simulink model "pos_8mot"  (R2021a)
settings: Solver=FixedStepDiscrete  StartTime=0.0  StopTime=inf  FixedStep=0.001  RelTol=1e-3  EnableMultiTasking=on
InitFcn:
  | load("rho_CommandCalib.mat");
  | run("importCmd.m")
model workspace (MAT data in the model file):
  positionCmd = [145.742 145.741 145.741 145.74 145.74 145.739 145.738 145.738 145.737 145.737 145.736 145.735 ... (560000 elements, 70000x8)]
  tempsTraj = [25 25 20]
values from neighbouring files (symbols this model uses):
  rho_CommandCalib = [325.033 325.033 325.033 325.033 325.033 325.033 325.033 325.033 325.033 325.033 325.033 325.033 ... (80000 elements, 10000x8)]    [rho_CommandCalib.mat]
undefined symbols (not defined in the file or in its folder): rho_CommandCircXY, rho_CommandCroixTilt, rho_CommandCroixXY, rho_CommandInclinaison, rho_CommandInclinaisonInterieure, rho_CommandPickAndPlace, rho_CommandPickAndPlaceTilt, rho_CommandPickAndPlaceVertical, rho_CommandPickAndPlaceX, rho_CommandSinusZ, rho_CommandSinusZ_decentree, rho_CommandTwist
libraries: xpcethercatlib x64, slrealtimeethercatlib x36, commutil2 x19, slrealtimeobsoletelib x7
(part 2 of 3)

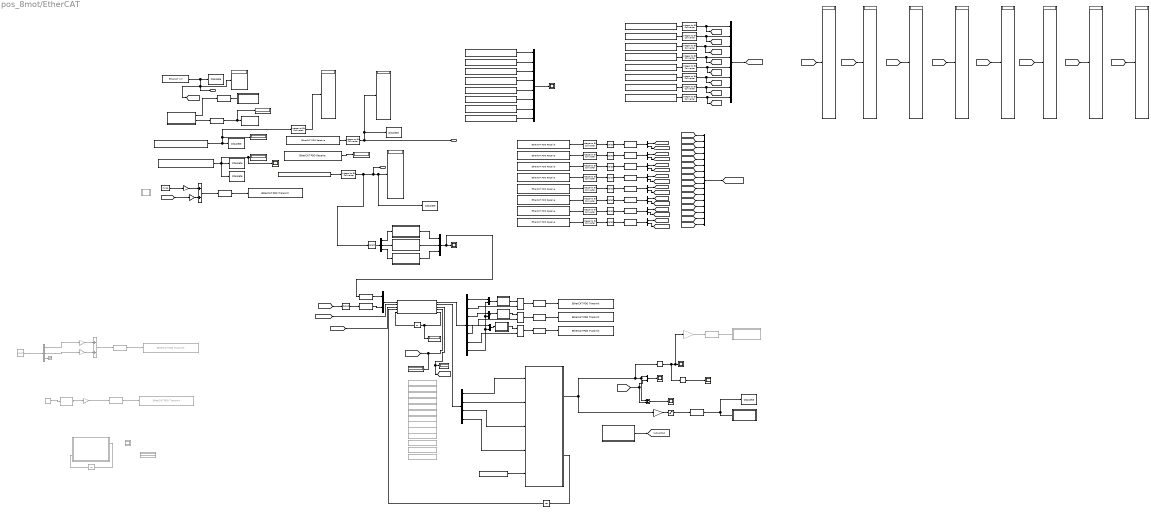
== system pos_8mot/EtherCAT ==
  note: Stand alone : PCI Bus 0 Slot 25, Otherwise : PCI Bus 3 Slot 0
  note: LinMot Warning Word
  note: Status Word from LinMot Drive
  note: Machine d'état
  note: Gestion des lumières
  note: Gestion des boutons
  note: Test 1 lumière clignotante
  note: Test 2 boutons 1 lumière
  note: Operation Enabled
      | Switch on Active
      | Operation Enabled
      | Fault
      | Voltage Enabled
      | Quick Stop
      | Switch on disabled
      | Warning
      | event Handler Active
      | Special Motion Active
      | Target Reached
      | Homed
      | Fatal Error
      | Motion Active
      | Range Indicator 1
      | Range Indicator 2
  note: 4688 = Standby
      | 4663 = Ready to go!!!
      | 536 = Fault
      | 4657 = Fault reset
  note: Set control word
  note: Operation Enabled
      | Switch on Active
      | Enable Operation
      | Fault
      | Voltage Enabled
      | Quick Stop
      | Switch on disabled
      | Warning
      | event Handler Active
      | Special Motion Active
      | Target Reached
      | Homed
      | Fatal Error
      | Motion Active
      | Range Indicator 1
      | Range Indicator 2
  note: Digital In X4.5
      | Digital In X4.6
      | Digital In X4.7
      | Digital In X4.8
      | Forced Bit Mask
      | Forced Bit Mask
      | empty
      | empty
      | empty
      | empty
      | empty
      | empty
      | empty
      | empty
      | empty
      | empty
  Activation1 : Subsystem
  Actual Motor Position : Subsystem
  Add : Sum
  Add1 : Sum  Commented=on
  Alimentation : Subsystem  Commented=on
      settings: OpenFcn=|
      | if strcmp(get_param([gcb '/Manual Switch'], 'sw'), '1')
      |   set_param([gcb '/Manual Switch'], 'sw', '0');
      |   set_param(gcb, 'MaskDisplay', 'fprintf(''ON'')','BackgroundColor','green');
      | else
      |   set_param([gcb '/Manual Switch'], 'sw', '1');
      |   set_param(gcb, 'MaskDisplay', 'fprintf(''OFF'')','BackgroundColor','red');
      | end
      mask Display: fprintf('OFF')
  Cast To Double{2..9} (8 alike) : DataTypeConversion  OutDataTypeStr=double
  Commande et réelle : Scope
  Constant : Constant  Commented=on  Value=[0.5 0]
  Constant1 : Constant  Commented=on  Value=rho_CommandPickAndPlace
  Constant10 : Constant  Commented=on  Value=rho_CommandInclinaisonInterieure
  Constant11 : Constant  Commented=on  Value=rho_CommandTwist
  Constant18 : Constant  Commented=on  Value=rho_CommandCalib
  Constant19 : Constant  Value=rho_CommandCalib
  Constant2 : Constant  Commented=on  Value=rho_CommandCroixTilt
  Constant21 : Constant  Commented=on  Value=rho_CommandSinusZ_decentree
  Constant22 : Constant  Commented=on  Value=rho_CommandPickAndPlaceVertical
  Constant3 : Constant  Commented=on  Value=rho_CommandPickAndPlaceX
  Constant4 : Constant  Commented=on  Value=rho_CommandSinusZ
  Constant5 : Constant  Commented=on  Value=rho_CommandCircXY
  Constant6 : Constant  Commented=on  Value=rho_CommandCroixXY
  Constant7 : Constant  Commented=on  Value=rho_CommandInclinaison
  Constant8 : Constant  Commented=on  Value=rho_CommandPickAndPlaceTilt
  Current Drive 1 : slrealtimeethercatlib/EtherCAT PDO Receive  Priority=2  sig_name=Drive 1 (C1150-DS-XC-0S).Cylic Mode Inputs.DemandCurrent  sig_offset=776  sig_type=int32  type_size=32  sig_dim=1  device_id=0  sample_time=0.001000
      settings: SourceProductBaseCode=XP
  Current Drive 10 : slrealtimeethercatlib/EtherCAT PDO Receive  Priority=2  sig_name=Drive 2 (C1150-DS-XC-0S).User Defined Inputs.Warn Word LinMot  sig_offset=1016  sig_type=uint16  type_size=16  sig_dim=1  device_id=0  sample_time=0.001000
      settings: SourceProductBaseCode=XP
  Current Drive 11 : slrealtimeethercatlib/EtherCAT PDO Receive  Priority=2  sig_name=Drive 3 (C1150-DS-XC-0S).User Defined Inputs.Warn Word LinMot  sig_offset=1176  sig_type=uint16  type_size=16  sig_dim=1  device_id=0  sample_time=0.001000
      settings: SourceProductBaseCode=XP
  Current Drive 12 : slrealtimeethercatlib/EtherCAT PDO Receive  Priority=2  sig_name=Drive 4 (C1150-DS-XC-0S).User Defined Inputs.Warn Word LinMot  sig_offset=1336  sig_type=uint16  type_size=16  sig_dim=1  device_id=0  sample_time=0.001000
      settings: SourceProductBaseCode=XP
  Current Drive 13 : slrealtimeethercatlib/EtherCAT PDO Receive  Priority=2  sig_name=Drive 5 (C1150-DS-XC-0S).User Defined Inputs.Warn Word LinMot  sig_offset=1496  sig_type=uint16  type_size=16  sig_dim=1  device_id=0  sample_time=0.001000
      settings: SourceProductBaseCode=XP
  Current Drive 14 : slrealtimeethercatlib/EtherCAT PDO Receive  Priority=2  sig_name=Drive 6 (C1150-DS-XC-0S).User Defined Inputs.Warn Word LinMot  sig_offset=1656  sig_type=uint16  type_size=16  sig_dim=1  device_id=0  sample_time=0.001000
      settings: SourceProductBaseCode=XP
  Current Drive 15 : slrealtimeethercatlib/EtherCAT PDO Receive  Priority=2  sig_name=Drive 7 (C1150-DS-XC-0S).User Defined Inputs.Warn Word LinMot  sig_offset=1816  sig_type=uint16  type_size=16  sig_dim=1  device_id=0  sample_time=0.001000
      settings: SourceProductBaseCode=XP
  Current Drive 16 : slrealtimeethercatlib/EtherCAT PDO Receive  Priority=2  sig_name=Drive 8 (C1150-DS-XC-0S).User Defined Inputs.Warn Word LinMot  sig_offset=1976  sig_type=uint16  type_size=16  sig_dim=1  device_id=0  sample_time=0.001000
      settings: SourceProductBaseCode=XP
  Current Drive 2 : slrealtimeethercatlib/EtherCAT PDO Receive  Priority=2  sig_name=Drive 2 (C1150-DS-XC-0S).Cylic Mode Inputs.DemandCurrent  sig_offset=952  sig_type=int32  type_size=32  sig_dim=1  device_id=0  sample_time=0.001000
      settings: SourceProductBaseCode=XP
  Current Drive 3 : slrealtimeethercatlib/EtherCAT PDO Receive  Priority=2  sig_name=Drive 3 (C1150-DS-XC-0S).Cylic Mode Inputs.DemandCurrent  sig_offset=1112  sig_type=int32  type_size=32  sig_dim=1  device_id=0  sample_time=0.001000
      settings: SourceProductBaseCode=XP
  Current Drive 4 : slrealtimeethercatlib/EtherCAT PDO Receive  Priority=2  sig_name=Drive 4 (C1150-DS-XC-0S).Cylic Mode Inputs.DemandCurrent  sig_offset=1272  sig_type=int32  type_size=32  sig_dim=1  device_id=0  sample_time=0.001000
      settings: SourceProductBaseCode=XP
  Current Drive 5 : slrealtimeethercatlib/EtherCAT PDO Receive  Priority=2  sig_name=Drive 5 (C1150-DS-XC-0S).Cylic Mode Inputs.DemandCurrent  sig_offset=1432  sig_type=int32  type_size=32  sig_dim=1  device_id=0  sample_time=0.001000
      settings: SourceProductBaseCode=XP
  Current Drive 6 : slrealtimeethercatlib/EtherCAT PDO Receive  Priority=2  sig_name=Drive 6 (C1150-DS-XC-0S).Cylic Mode Inputs.DemandCurrent  sig_offset=1592  sig_type=int32  type_size=32  sig_dim=1  device_id=0  sample_time=0.001000
      settings: SourceProductBaseCode=XP
  Current Drive 7 : slrealtimeethercatlib/EtherCAT PDO Receive  Priority=2  sig_name=Drive 7 (C1150-DS-XC-0S).Cylic Mode Inputs.DemandCurrent  sig_offset=1752  sig_type=int32  type_size=32  sig_dim=1  device_id=0  sample_time=0.001000
      settings: SourceProductBaseCode=XP
  Current Drive 8 : slrealtimeethercatlib/EtherCAT PDO Receive  Priority=2  sig_name=Drive 8 (C1150-DS-XC-0S).Cylic Mode Inputs.DemandCurrent  sig_offset=1912  sig_type=int32  type_size=32  sig_dim=1  device_id=0  sample_time=0.001000
      settings: SourceProductBaseCode=XP
  Current Drive 9 : slrealtimeethercatlib/EtherCAT PDO Receive  Priority=2  sig_name=Drive 1 (C1150-DS-XC-0S).User Defined Inputs.Warn Word LinMot  sig_offset=856  sig_type=uint16  type_size=16  sig_dim=1  device_id=0  sample_time=0.001000
      settings: SourceProductBaseCode=XP
  Data Type Conversion : DataTypeConversion  OutDataTypeStr=int32
  Data Type Conversion{1,3,8..10} (5 alike) : DataTypeConversion  OutDataTypeStr=uint16
  Data Type Conversion11 : DataTypeConversion  Commented=on  OutDataTypeStr=int32
  Data Type Conversion2 : DataTypeConversion  OutDataTypeStr=int8
  Data Type Conversion4 : DataTypeConversion  Commented=on  OutDataTypeStr=uint16
  Data Type Conversion5 : DataTypeConversion  Commented=on  OutDataTypeStr=uint16
  Data Type Conversion6 : DataTypeConversion  OutDataTypeStr=double
  Data Type Conversion7 : DataTypeConversion  OutDataTypeStr=double
  Demux : Demux  Commented=on  Outputs=3
  Demux1 : Demux  Outputs=3
  Demux{4..11} (8 alike) : Demux  Outputs=2
  Demux2 : Demux  Outputs=7
  Demux3 : Demux
  Digital In Word form Linmot UPID : slrealtimeethercatlib/EtherCAT PDO Receive  Priority=2  sig_name=Drive 1 (C1150-DS-XC-0S).User Defined Inputs.Digital Input Word  sig_offset=824  sig_type=uint16  type_size=16  sig_dim=1  device_id=0  sample_time=0.001000
      settings: SourceProductBaseCode=XP
  Digital Output Word : slrealtimeethercatlib/EtherCAT PDO Transmit  Priority=3  sig_name=Drive 1 (C1150-DS-XC-0S).User Defined Outputs.Digital Output Word  sig_offset=760  sig_type=uint16  type_size=16  sig_dim=1  device_id=0  sample_time=0.001000
      settings: SourceProductBaseCode=XP
  Digital Output Word1 : slrealtimeethercatlib/EtherCAT PDO Transmit  Priority=3  Commented=on  sig_name=Drive 2 (C1150-DS-XC-0S).User Defined Outputs.Digital Output Word  sig_offset=920  sig_type=uint16  type_size=16  sig_dim=1  device_id=0  sample_time=0.001000
      settings: SourceProductBaseCode=XP
  Digital Output Word2 : slrealtimeethercatlib/EtherCAT PDO Transmit  Priority=3  Commented=on  sig_name=Drive 2 (C1150-DS-XC-0S).User Defined Outputs.Digital Output Word  sig_offset=920  sig_type=uint16  type_size=16  sig_dim=1  device_id=0  sample_time=0.001000
      settings: SourceProductBaseCode=XP
  Digital Output Word3 : slrealtimeethercatlib/EtherCAT PDO Transmit  Priority=3  sig_name=Drive 2 (C1150-DS-XC-0S).User Defined Outputs.Digital Output Word  sig_offset=936  sig_type=uint16  type_size=16  sig_dim=1  device_id=0  sample_time=0.001000
      settings: SourceProductBaseCode=XP
  Digital Output Word4 : slrealtimeethercatlib/EtherCAT PDO Transmit  Priority=3  sig_name=Drive 3 (C1150-DS-XC-0S).User Defined Outputs.Digital Output Word  sig_offset=1096  sig_type=uint16  type_size=16  sig_dim=1  device_id=0  sample_time=0.001000
      settings: SourceProductBaseCode=XP
  Digital Output Word5 : slrealtimeethercatlib/EtherCAT PDO Transmit  Priority=3  sig_name=Drive 4 (C1150-DS-XC-0S).User Defined Outputs.Digital Output Word  sig_offset=1256  sig_type=uint16  type_size=16  sig_dim=1  device_id=0  sample_time=0.001000
      settings: SourceProductBaseCode=XP
  Display{,1..4,6..14} (14 alike) : Display
  Display5 : Display  Commented=on
  Erreur : Scope
  "EtherCAT Init " : slrealtimeethercatlib/EtherCAT Init  Priority=0  config_file=U:\Maitrise\Planification de trajectoire\TwinCAT\8motor_pos_control_IO\8mot_poscont_IO_ENI_V2.xml  device_id=0  pci_bus=0  pci_slot=0  pci_function=0  portnum=1  initstate=2  dctuning=0  enaDebug=0  enaDC=on  errLink=off  masterDbg=off  stateChgDbg=off  baseClock=off  masterCfg=off  logFile='c:\dbglog.txt'  sample_time=0.001000  DCMode=2
      settings: SourceProductBaseCode=XP
  Gain : Gain  Gain=2^0
  Gain1 : Gain  Gain=2^1
  Gain2 : Gain  Commented=on  Gain=2^0
  Gain3 : Gain  Commented=on  Gain=2^1
  Gain4 : Gain  Commented=on  Gain=2^0
  Integer to Bit Converter{,1..18} (19 alike) : commutil2/Integer to Bit Converter  nbits=16  signedInputValues=Unsigned  bitOrder=LSB first  outDtype=Inherit via internal rule
  LOG_Acceleration : Derivative
  LOG_Current : Mux  Inputs=8
  LOG_Erreur : Sum  Inputs=+-
  LOG_Vitesse : Derivative
  MATLAB Function : MATLAB Function  Commented=on  TreatAsAtomicUnit=on
  MATLAB Function1 : MATLAB Function  TreatAsAtomicUnit=on
  MATLAB Function2 : MATLAB Function  Commented=on  TreatAsAtomicUnit=on
  MATLAB Function3 : MATLAB Function  TreatAsAtomicUnit=on
  MATLAB Function4 : MATLAB Function  TreatAsAtomicUnit=on
  MATLAB Function5 : MATLAB Function  TreatAsAtomicUnit=on
  MATLAB Function6 : MATLAB Function  TreatAsAtomicUnit=on
  MATLAB Function7 : MATLAB Function  TreatAsAtomicUnit=on
  MATLAB Function8 : MATLAB Function  TreatAsAtomicUnit=on
  MATLAB Function9 : MATLAB Function  TreatAsAtomicUnit=on
  Matrix Multiply : Product  Multiplication=Matrix(*)
  Matrix Multiply1 : Product  Multiplication=Matrix(*)
  Matrix Multiply2 : Product  Multiplication=Matrix(*)
  Mode : Display
  Mode Selection : Display
  Mode of Operation Display : slrealtimeethercatlib/EtherCAT PDO Receive  Priority=2  sig_name=Drive 7 (C1150-DS-XC-0S).Cylic Mode Inputs.Mode of Operation display  sig_offset=1784  sig_type=int8  type_size=8  sig_dim=1  device_id=0  sample_time=0.001000
      settings: SourceProductBaseCode=XP
  Mux : Mux  Inputs=3
  Mux{1..5} (5 alike) : Mux  Inputs=2
  Mux8 : Mux  Inputs=16
  Position : Display
  Position Actual Value : slrealtimeethercatlib/EtherCAT PDO Receive  Priority=2  sig_name=Drive 7 (C1150-DS-XC-0S).Cylic Mode Inputs.Position actual value (units)  sig_offset=1688  sig_type=int32  type_size=32  sig_dim=1  device_id=0  sample_time=0.001000
      settings: SourceProductBaseCode=XP
  Pulse WatchDog : DiscretePulseGenerator  PulseType=Time based  Period=0.1  PulseWidth=50
  Saturation1 : Saturate  UpperLimit=3250000  LowerLimit=10000
  Scope : Scope  Commented=on
  Scope Position : Scope
  "Scope " : slrealtimeobsoletelib/Obsolete  ObsoleteBlock=slrtlib/Displays and Logging/Scope  ObsoleteParameters=|  NumInports=1  NumOutports=0
      | ContentPreviewEnabled:  off
      | scopeno:  1
      | scopetype:  Target
      | autostart:  on
      | viewmode:  Numerical
      | formatstr:  '%6.0f,%6.0f,%6.0f,%6.0f,%6.0f,%6.0f'
      | grid:  on
      | ylimits:  [0,0]
      | nosamples:  3
      | noprepostsamples:  0
      | interleave:  1
      | triggermode:  FreeRun
      | triggersignal:  1
      | trigsignalfromport:  off
      | triggerlevel:  0.0
      | triggerslope:  Either
      | triggerscope:  1
      | triggersample:  0
      | filename:  data.dat
      | mode:  Lazy
      | writesize:  512
      | autorestart:  off
      | dynamicfilemode:  off
      | maxwritefilesize:  512*1024^2
      settings: SourceProductBaseCode=XP
  Scope 1 : slrealtimeobsoletelib/Obsolete  ObsoleteBlock=slrtlib/Displays and Logging/Scope  ObsoleteParameters=|  NumInports=1  NumOutports=0
      | ContentPreviewEnabled:  off
      | scopeno:  3
      | scopetype:  Target
      | autostart:  on
      | viewmode:  Numerical
      | formatstr:  '%15.6f'
      | grid:  on
      | ylimits:  [0,0]
      | nosamples:  3
      | noprepostsamples:  0
      | interleave:  1
      | triggermode:  FreeRun
      | triggersignal:  1
      | trigsignalfromport:  off
      | triggerlevel:  0.0
      | triggerslope:  Either
      | triggerscope:  1
      | triggersample:  0
      | filename:  data.dat
      | mode:  Lazy
      | writesize:  512
      | autorestart:  off
      | dynamicfilemode:  off
      | maxwritefilesize:  512*1024^2
      settings: SourceProductBaseCode=XP
  Scope 2 : slrealtimeobsoletelib/Obsolete  ObsoleteBlock=slrtlib/Displays and Logging/Scope  ObsoleteParameters=|  NumInports=1  NumOutports=0
      | ContentPreviewEnabled:  off
      | scopeno:  4
      | scopetype:  Target
      | autostart:  on
      | viewmode:  Graphical sliding
      | formatstr:  '%15.6f'
      | grid:  on
      | ylimits:  [-1000000,1000000]
      | nosamples:  2000
      | noprepostsamples:  0
      | interleave:  1
      | triggermode:  FreeRun
      | triggersignal:  1
      | trigsignalfromport:  off
      | triggerlevel:  0.0
      | triggerslope:  Either
      | triggerscope:  1
      | triggersample:  0
      | filename:  data.dat
      | mode:  Lazy
      | writesize:  512
      | autorestart:  off
      | dynamicfilemode:  off
      | maxwritefilesize:  512*1024^2
      settings: SourceProductBaseCode=XP
  Scope 3 : slrealtimeobsoletelib/Obsolete  ObsoleteBlock=slrtlib/Displays and Logging/Scope  ObsoleteParameters=|  NumInports=1  NumOutports=0
      | ContentPreviewEnabled:  off
      | scopeno:  2
      | scopetype:  Target
      | autostart:  on
      | viewmode:  Graphical sliding
      | formatstr:  '%15.6f'
      | grid:  on
      | ylimits:  [0,0]
      | nosamples:  1000
      | noprepostsamples:  0
      | interleave:  1
      | triggermode:  FreeRun
      | triggersignal:  1
      | trigsignalfromport:  off
      | triggerlevel:  0.0
      | triggerslope:  Either
      | triggerscope:  1
      | triggersample:  0
      | filename:  data.dat
      | mode:  Lazy
      | writesize:  512
      | autorestart:  off
      | dynamicfilemode:  off
      | maxwritefilesize:  512*1024^2
      settings: SourceProductBaseCode=XP
  Scope 4 : slrealtimeobsoletelib/Obsolete  ObsoleteBlock=slrtlib/Displays and Logging/Scope  ObsoleteParameters=|  NumInports=1  NumOutports=0
      | ContentPreviewEnabled:  off
      | scopeno:  5
      | scopetype:  Target
      | autostart:  on
      | viewmode:  Numerical
      | formatstr:  '%15.6f'
      | grid:  on
      | ylimits:  [0,0]
      | nosamples:  3
      | noprepostsamples:  0
      | interleave:  1
      | triggermode:  FreeRun
      | triggersignal:  1
      | trigsignalfromport:  off
      | triggerlevel:  0.0
      | triggerslope:  Either
      | triggerscope:  1
      | triggersample:  0
      | filename:  data.dat
      | mode:  Lazy
      | writesize:  512
      | autorestart:  off
      | dynamicfilemode:  off
      | maxwritefilesize:  512*1024^2
      settings: SourceProductBaseCode=XP
  Scope 5 : slrealtimeobsoletelib/Obsolete  ObsoleteBlock=slrtlib/Displays and Logging/Scope  ObsoleteParameters=|  NumInports=1  NumOutports=0
      | ContentPreviewEnabled:  off
      | scopeno:  6
      | scopetype:  Target
      | autostart:  on
      | viewmode:  Numerical
      | formatstr:  'Digital In X4.5 %1.0f, Digital In X4.6 %1.0f, Digital In X4.7 %1.0f, Digital In X4.8 %1.0f, Forced Bit Mask %1.0f, Forced Bit Mask %1.0f'
      | grid:  on
      | ylimits:  [0,0]
      | nosamples:  3
      | noprepostsamples:  0
      | interleave:  1
      | triggermode:  FreeRun
      | triggersignal:  1
      | trigsignalfromport:  off
      | triggerlevel:  0.0
      | triggerslope:  Either
      | triggerscope:  1
      | triggersample:  0
      | filename:  data.dat
      | mode:  Lazy
      | writesize:  512
      | autorestart:  off
      | dynamicfilemode:  off
      | maxwritefilesize:  512*1024^2
      settings: SourceProductBaseCode=XP
  Scope 6 : slrealtimeobsoletelib/Obsolete  ObsoleteBlock=slrtlib/Displays and Logging/Scope  ObsoleteParameters=|  NumInports=1  NumOutports=0
      | ContentPreviewEnabled:  off
      | scopeno:  7
      | scopetype:  Target
      | autostart:  on
      | viewmode:  Numerical
      | formatstr:  'Operation Enabled %1.0f, Switch on Active %1.0f, Enable Operation %1.0f, Fault %1.0f, Voltage Enabled %1.0f, Quick Stop %1.0f, Switch on disabled %1.0f, Warning %1.0f, event Handler Active %1.0f, Special Motion Active %1.0f, target Reached %1.0f, Homed %1.0f, Fatal Error %1.0f, Motion Active %1.0f, Range Indicator 1 %1.0f, Range Indicator 2 %1.0f'
      | grid:  on
      | ylimits:  [0,0]
      | nosamples:  3
      | noprepostsamples:  0
      | interleave:  1
      | triggermode:  FreeRun
      | triggersignal:  1
      | trigsignalfromport:  off
      | triggerlevel:  0.0
      | triggerslope:  Either
      | triggerscope:  1
      | triggersample:  0
      | filename:  data.dat
      | mode:  Lazy
      | writesize:  512
      | autorestart:  off
      | dynamicfilemode:  off
      | maxwritefilesize:  512*1024^2
      settings: SourceProductBaseCode=XP
  Scope{1..2,4..5} (4 alike) : Scope
  Selector : Selector  Commented=on  InputPortWidth=16  IndexOptions=Index vector (dialog)  Indices=[1 2 3]  OutputSizes=1
  Selector1 : Selector  InputPortWidth=16  IndexOptions=Index vector (dialog)  Indices=[1 2 3]  OutputSizes=1
  Selector{4..11} (8 alike) : Selector  InputPortWidth=16  IndexOptions=Index vector (dialog)  Indices=[4 12]  OutputSizes=1
  Selector2 : Selector  InputPortWidth=6  IndexOptions=Index vector (dialog)  Indices=[2]  OutputSizes=1
  Send Control Word : Subsystem
  Send Position : Subsystem
  Send mode of opreation : Subsystem
  Send velocity : Subsystem  Commented=on
  State : Display
  StatuWord from Linmot UPID : slrealtimeethercatlib/EtherCAT PDO Receive  Priority=2  sig_name=Drive 7 (C1150-DS-XC-0S).User Defined Inputs.StatusWord Linmot  sig_offset=1800  sig_type=uint16  type_size=16  sig_dim=1  device_id=0  sample_time=0.001000
      settings: SourceProductBaseCode=XP
  StatuWord from Linmot UPID1 : slrealtimeethercatlib/EtherCAT PDO Receive  Priority=2  sig_name=Drive 1 (C1150-DS-XC-0S).User Defined Inputs.StatusWord Linmot  sig_offset=840  sig_type=uint16  type_size=16  sig_dim=1  device_id=0  sample_time=0.001000
      settings: SourceProductBaseCode=XP
  StatuWord from Linmot UPID2 : slrealtimeethercatlib/EtherCAT PDO Receive  Priority=2  sig_name=Drive 2 (C1150-DS-XC-0S).User Defined Inputs.StatusWord Linmot  sig_offset=1000  sig_type=uint16  type_size=16  sig_dim=1  device_id=0  sample_time=0.001000
      settings: SourceProductBaseCode=XP
  StatuWord from Linmot UPID3 : slrealtimeethercatlib/EtherCAT PDO Receive  Priority=2  sig_name=Drive 3 (C1150-DS-XC-0S).User Defined Inputs.StatusWord Linmot  sig_offset=1160  sig_type=uint16  type_size=16  sig_dim=1  device_id=0  sample_time=0.001000
      settings: SourceProductBaseCode=XP
  StatuWord from Linmot UPID4 : slrealtimeethercatlib/EtherCAT PDO Receive  Priority=2  sig_name=Drive 4 (C1150-DS-XC-0S).User Defined Inputs.StatusWord Linmot  sig_offset=1320  sig_type=uint16  type_size=16  sig_dim=1  device_id=0  sample_time=0.001000
      settings: SourceProductBaseCode=XP
  StatuWord from Linmot UPID5 : slrealtimeethercatlib/EtherCAT PDO Receive  Priority=2  sig_name=Drive 5 (C1150-DS-XC-0S).User Defined Inputs.StatusWord Linmot  sig_offset=1480  sig_type=uint16  type_size=16  sig_dim=1  device_id=0  sample_time=0.001000
      settings: SourceProductBaseCode=XP
  StatuWord from Linmot UPID6 : slrealtimeethercatlib/EtherCAT PDO Receive  Priority=2  sig_name=Drive 6 (C1150-DS-XC-0S).User Defined Inputs.StatusWord Linmot  sig_offset=1640  sig_type=uint16  type_size=16  sig_dim=1  device_id=0  sample_time=0.001000
      settings: SourceProductBaseCode=XP
  StatuWord from Linmot UPID7 : slrealtimeethercatlib/EtherCAT PDO Receive  Priority=2  sig_name=Drive 7 (C1150-DS-XC-0S).User Defined Inputs.StatusWord Linmot  sig_offset=1800  sig_type=uint16  type_size=16  sig_dim=1  device_id=0  sample_time=0.001000
      settings: SourceProductBaseCode=XP
  StatuWord from Linmot UPID8 : slrealtimeethercatlib/EtherCAT PDO Receive  Priority=2  sig_name=Drive 8 (C1150-DS-XC-0S).User Defined Inputs.StatusWord Linmot  sig_offset=1960  sig_type=uint16  type_size=16  sig_dim=1  device_id=0  sample_time=0.001000
      settings: SourceProductBaseCode=XP
  StatusWord : slrealtimeethercatlib/EtherCAT PDO Receive  Priority=2  sig_name=Drive 7 (C1150-DS-XC-0S).Cylic Mode Inputs.Statusword  sig_offset=1672  sig_type=uint16  type_size=16  sig_dim=1  device_id=0  sample_time=0.001000
      settings: SourceProductBaseCode=XP
  Terminator : Terminator  Commented=on
  Unit Delay : UnitDelay  Commented=on  SampleTime=-1  HasFrameUpgradeWarning=on
  Unit Delay1 : UnitDelay  SampleTime=-1  HasFrameUpgradeWarning=on
  Unit Delay2 : UnitDelay  SampleTime=-1  HasFrameUpgradeWarning=on
  Vector Concatenate : Concatenate  NumInputs=8  Mode=Multidimensional array  ConcatenateDimension=2
  mm to um : Gain  Commented=on  Gain=10000
  signaux : Display
  to linmot unit : Gain  Gain=10000
  ECAT_status : Outport
  SW_linmot : Outport  Port=2
  Digital_IN : Outport  Port=3
  tag scope: modeSelection=global
  wires:
  Activation1/2(ControlWord) -> Data Type Conversion1/1
  Data Type Conversion1/1 -> Send Control Word/1(In1), Display2/1
  Data Type Conversion/1 -> Send Position/1(Commanded Position), Scope 3/1  "Commanded Position"
  StatusWord/1 -> Integer to Bit Converter/1, Display/1, Scope 1/1  "Status word"
  Position Actual Value/1 -> Scope 4/1, Scope Position/1, Position/1, Scope 2/1  "Actual Position"
  Saturation1/1 -> Data Type Conversion/1
  Mode of Operation Display/1 -> Mode/1  "Status word"
  Integer to Bit Converter/1 -> Display3/1
  to linmot unit/1 -> Saturation1/1
  Digital In Word form Linmot UPID/1 -> Integer to Bit Converter1/1  "digital"
  Integer to Bit Converter1/1 -> Selector1/1, Digital_IN/1, Scope 5/1, signaux/1
  StatuWord from Linmot UPID/1 -> Integer to Bit Converter2/1  "bouton"
  Integer to Bit Converter2/1 -> SW_linmot/1, Scope 6/1, Display4/1
  Gain1/1 -> Add/2
  Gain/1 -> Add/1
  Pulse WatchDog/1 -> Gain/1
  Add/1 -> Data Type Conversion3/1
  Data Type Conversion3/1 -> Digital Output Word/1
  Data Type Conversion2/1 -> Send mode of opreation/1(In1)
  Activation1/1(mode of operation) -> Data Type Conversion2/1
  Data Type Conversion4/1 -> Digital Output Word1/1
  Demux/2 -> Gain3/1
  Gain2/1 -> Add1/1
  Gain3/1 -> Add1/2
  Demux/1 -> Gain2/1
  Add1/1 -> Data Type Conversion4/1
  Selector/1 -> Demux/1
  Demux/3 -> Terminator/1
  MATLAB Function/1(y) -> Gain4/1
  Gain4/1 -> Data Type Conversion5/1
  Data Type Conversion5/1 -> Digital Output Word2/1
  MATLAB Function2/1(new_state) -> Unit Delay/1
  Unit Delay/1 -> MATLAB Function2/2(state)
  Mux/1 -> Data Type Conversion7/1, Scope1/1
  MATLAB Function1/1(isPressed) -> Mux/1
  MATLAB Function3/1(isPressed) -> Mux/2
  MATLAB Function4/1(isPressed) -> Mux/3
  Selector1/1 -> Demux1/1
  Demux1/2 -> MATLAB Function3/1(buttonState)
  Demux1/1 -> MATLAB Function1/1(buttonState)
  Demux1/3 -> MATLAB Function4/1(buttonState)
  "EtherCAT Init "/1 -> [ECAT_Status], ECAT_status/1, Display1/1, "Scope "/1
  [ECAT_Status] -> Selector2/1
  Mux1/1 -> MATLAB Function5/1(inputs)
  MATLAB Function5/5(new_state) -> State/1, Unit Delay1/1
  Unit Delay1/1 -> MATLAB Function5/5(state)
  Selector2/1 -> Data Type Conversion6/1
  Data Type Conversion6/1 -> Mux1/2
  Data Type Conversion7/1 -> Mux1/1
  Data Type Conversion10/1 -> Digital Output Word5/1
  Data Type Conversion9/1 -> Digital Output Word4/1
  Data Type Conversion8/1 -> Digital Output Word3/1
  Matrix Multiply2/1 -> Data Type Conversion8/1
  Matrix Multiply1/1 -> Data Type Conversion9/1
  Matrix Multiply/1 -> Data Type Conversion10/1
  MATLAB Function5/1(outputs_LED) -> Demux2/1
  Constant/1 -> MATLAB Function/1(u)
  MATLAB Function8/1(y) -> Matrix Multiply/1
  MATLAB Function7/1(y) -> Matrix Multiply1/1
  MATLAB Function6/1(y) -> Matrix Multiply2/1
  Demux2/2 -> Matrix Multiply2/2
  Demux2/4 -> Matrix Multiply1/2
  Demux2/6 -> Matrix Multiply/2
  Demux2/1 -> Mux2/1
  Demux2/3 -> Mux3/1
  Demux2/5 -> Mux4/1
  Mux2/1 -> MATLAB Function6/1(u)
  Demux2/7 -> Mux4/2, Mux3/2, Mux2/2
  Mux4/1 -> MATLAB Function8/1(u)
  Mux3/1 -> MATLAB Function7/1(u)
  MATLAB Function5/2(outputs_traj) -> Demux3/1
  MATLAB Function5/3(selectionMode) -> [modeSelection], Mode Selection/1
  Demux3/1 -> MATLAB Function9/1(trajectorySelector)
  Demux3/2 -> MATLAB Function9/2(pause)
  Demux3/3 -> MATLAB Function9/3(stopAtEnd)
  Demux3/4 -> MATLAB Function9/4(waitForActivation)
  Constant19/1 -> MATLAB Function9/5(position_from_gabarit_to_standby)
  MATLAB Function9/2(isCompleted) -> Unit Delay2/1
  Unit Delay2/1 -> MATLAB Function5/4(isCompleted)
  Mux5/1 -> Commande et réelle/1
  LOG_Erreur/1 -> Erreur/1
  [ActualPos] -> Mux5/2, LOG_Erreur/2
  MATLAB Function5/4(motorPower) -> Display6/1, [motorPower]
  [StatusWord_LinMot] -> MATLAB Function5/2(statusWordLinMot)
  [motorPower] -> Gain1/1
  MATLAB Function9/1(target) -> LOG_Vitesse/1, Mux5/1, LOG_Erreur/1, to linmot unit/1
  Actual Motor Position/1(Actual Position) -> [ActualPos]
  Current Drive 8/1 -> LOG_Current/8
  Current Drive 6/1 -> LOG_Current/6
  Current Drive 7/1 -> LOG_Current/7
  Current Drive 5/1 -> LOG_Current/5
  Current Drive 4/1 -> LOG_Current/4
  Current Drive 3/1 -> LOG_Current/3
  Current Drive 2/1 -> LOG_Current/2
  Current Drive 1/1 -> LOG_Current/1
  LOG_Current/1 -> Scope4/1
  LOG_Vitesse/1 -> LOG_Acceleration/1, mm to um/1, Scope5/1
  Data Type Conversion11/1 -> Send velocity/1(Command velocity)  "Commanded Velocity"
  mm to um/1 -> Data Type Conversion11/1
  LOG_Acceleration/1 -> Scope2/1
  StatuWord from Linmot UPID1/1 -> Integer to Bit Converter3/1  "bouton"
  StatuWord from Linmot UPID2/1 -> Integer to Bit Converter4/1  "bouton"
  StatuWord from Linmot UPID3/1 -> Integer to Bit Converter5/1  "bouton"
  StatuWord from Linmot UPID4/1 -> Integer to Bit Converter6/1  "bouton"
  StatuWord from Linmot UPID5/1 -> Integer to Bit Converter7/1  "bouton"
  StatuWord from Linmot UPID6/1 -> Integer to Bit Converter8/1  "bouton"
  StatuWord from Linmot UPID7/1 -> Integer to Bit Converter9/1  "bouton"
  StatuWord from Linmot UPID8/1 -> Integer to Bit Converter10/1  "bouton"
  Selector4/1 -> Cast To Double2/1
  Selector5/1 -> Cast To Double3/1
  Selector6/1 -> Cast To Double4/1
  Selector7/1 -> Cast To Double5/1
  Selector8/1 -> Cast To Double6/1
  Selector9/1 -> Cast To Double7/1
  Selector10/1 -> Cast To Double8/1
  Selector11/1 -> Cast To Double9/1
  Integer to Bit Converter3/1 -> Selector4/1
  Integer to Bit Converter4/1 -> Selector5/1
  Integer to Bit Converter5/1 -> Selector6/1
  Integer to Bit Converter6/1 -> Selector7/1
  Integer to Bit Converter7/1 -> Selector8/1
  Integer to Bit Converter8/1 -> Selector9/1
  Integer to Bit Converter9/1 -> Selector10/1
  Integer to Bit Converter10/1 -> Selector11/1
  Cast To Double2/1 -> Demux4/1
  Cast To Double3/1 -> Demux5/1
  Cast To Double4/1 -> Demux6/1
  Cast To Double5/1 -> Demux7/1
  Cast To Double6/1 -> Demux8/1
  Cast To Double7/1 -> Demux9/1
  Cast To Double8/1 -> Demux10/1
  Cast To Double9/1 -> Demux11/1
  Demux4/1 -> [faultDrive1]
  Demux4/2 -> [isHomedDrive1]
  Demux5/1 -> [faultDrive2]
  Demux5/2 -> [isHomedDrive2]
  Demux6/1 -> [faultDrive3]
  Demux6/2 -> [isHomedDrive3]
  Demux7/1 -> [faultDrive4]
  Demux7/2 -> [isHomedDrive4]
  Demux8/1 -> [faultDrive5]
  Demux8/2 -> [isHomedDrive5]
  Demux9/1 -> [faultDrive6]
  Demux9/2 -> [isHomedDrive6]
  Demux10/1 -> [faultDrive7]
  Demux10/2 -> [isHomedDrive7]
  Demux11/1 -> [faultDrive8]
  Demux11/2 -> [isHomedDrive8]
  [faultDrive6] -> Mux8/6
  [faultDrive1] -> Mux8/1
  [faultDrive2] -> Mux8/2
  [faultDrive3] -> Mux8/3
  [faultDrive4] -> Mux8/4
  [faultDrive5] -> Mux8/5
  [faultDrive7] -> Mux8/7
  [faultDrive8] -> Mux8/8
  [isHomedDrive1] -> Mux8/9
  [isHomedDrive2] -> Mux8/10
  [isHomedDrive3] -> Mux8/11
  [isHomedDrive4] -> Mux8/12
  [isHomedDrive5] -> Mux8/13
  [isHomedDrive6] -> Mux8/14
  [isHomedDrive7] -> Mux8/15
  [isHomedDrive8] -> Mux8/16
  Mux8/1 -> [StatusWord_LinMot]
  Current Drive 9/1 -> Integer to Bit Converter11/1
  Current Drive 10/1 -> Integer to Bit Converter12/1
  Current Drive 11/1 -> Integer to Bit Converter13/1
  Current Drive 12/1 -> Integer to Bit Converter14/1
  Current Drive 13/1 -> Integer to Bit Converter15/1
  Current Drive 14/1 -> Integer to Bit Converter16/1
  Current Drive 15/1 -> Integer to Bit Converter17/1
  Current Drive 16/1 -> Integer to Bit Converter18/1
  Integer to Bit Converter11/1 -> [warnWord1], Vector Concatenate/1
  Integer to Bit Converter12/1 -> [warnWord2], Vector Concatenate/2
  Integer to Bit Converter13/1 -> [warnWord3], Vector Concatenate/3
  Integer to Bit Converter14/1 -> [warnWord4], Vector Concatenate/4
  Integer to Bit Converter15/1 -> [warnWord5], Vector Concatenate/5
  Integer to Bit Converter16/1 -> [warnWord6], Vector Concatenate/6
  Integer to Bit Converter18/1 -> [warnWord8], Vector Concatenate/8
  Vector Concatenate/1 -> [WarnWord]
  [WarnWord] -> MATLAB Function5/3(warnWord)
  Integer to Bit Converter17/1 -> [warnWord7], Vector Concatenate/7
  [warnWord1] -> Display7/1
  [warnWord2] -> Display8/1
  [warnWord3] -> Display9/1
  [warnWord4] -> Display10/1
  [warnWord5] -> Display12/1
  [warnWord6] -> Display13/1
  [warnWord7] -> Display14/1
  [warnWord8] -> Display11/1

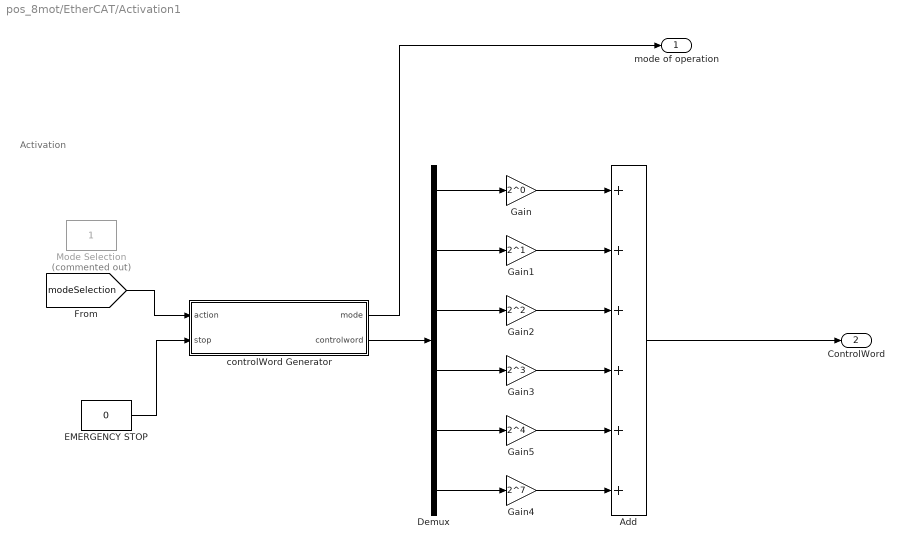
== system pos_8mot/EtherCAT/Activation1 ==
  note: Activation
  Add : Sum  Inputs=++++++
  Demux : Demux  Outputs=6
  EMERGENCY STOP : Constant  Value=0
  Gain : Gain  Gain=2^0
  Gain1 : Gain  Gain=2^1
  Gain2 : Gain  Gain=2^2
  Gain3 : Gain  Gain=2^3
  Gain4 : Gain  Gain=2^7
  Gain5 : Gain  Gain=2^4
  Mode Selection : Constant  Commented=on
  controlWord Generator : MATLAB Function  TreatAsAtomicUnit=on
  mode of operation : Outport
  ControlWord : Outport  Port=2
  wires:
  Add/1 -> ControlWord/1
  EMERGENCY STOP/1 -> controlWord Generator/2(stop)
  Demux/1 -> Gain/1
  Gain1/1 -> Add/2
  Gain3/1 -> Add/4
  Gain4/1 -> Add/6
  Demux/5 -> Gain5/1
  controlWord Generator/2(controlword) -> Demux/1
  Demux/2 -> Gain1/1
  Demux/6 -> Gain4/1
  Demux/3 -> Gain2/1
  Gain5/1 -> Add/5
  Gain/1 -> Add/1
  Gain2/1 -> Add/3
  Demux/4 -> Gain3/1
  controlWord Generator/1(mode) -> mode of operation/1
  [modeSelection] -> controlWord Generator/1(action)

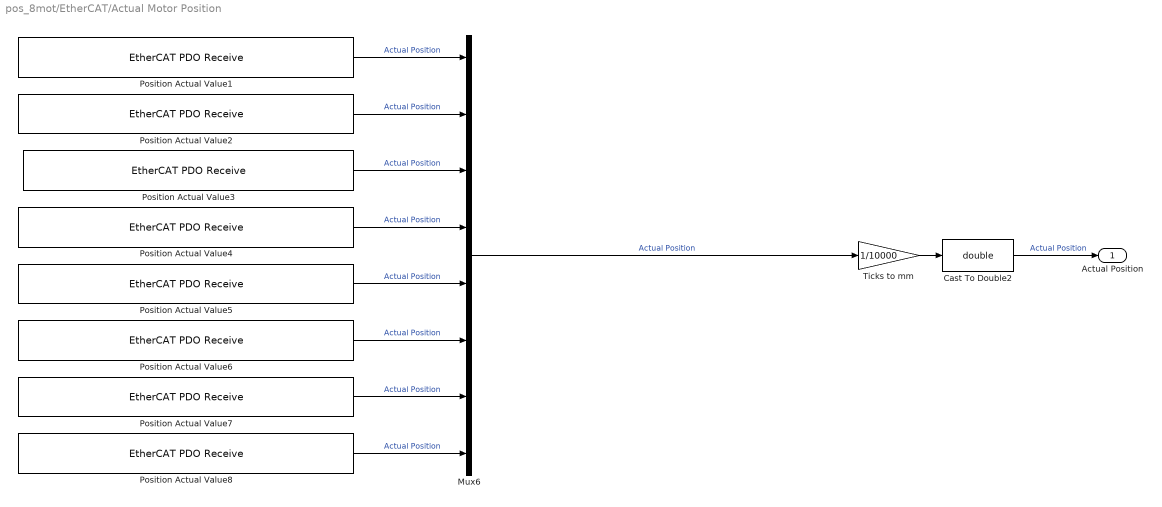
== system pos_8mot/EtherCAT/Actual Motor Position ==
  Cast To Double2 : DataTypeConversion  OutDataTypeStr=double
  Mux6 : Mux  Inputs=8
  Position Actual Value1 : xpcethercatlib/EtherCAT PDO Receive  Priority=2  sig_name=Drive 1 (C1150-DS-XC-0S).Cylic Mode Inputs.Position actual value (units)  sig_offset=712  sig_type=int32  type_size=32  sig_dim=1  device_id=0  sample_time=0.001000
      settings: SourceProductBaseCode=XP
  Position Actual Value2 : xpcethercatlib/EtherCAT PDO Receive  Priority=2  sig_name=Drive 2 (C1150-DS-XC-0S).Cylic Mode Inputs.Position actual value (units)  sig_offset=888  sig_type=int32  type_size=32  sig_dim=1  device_id=0  sample_time=0.001000
      settings: SourceProductBaseCode=XP
  Position Actual Value3 : xpcethercatlib/EtherCAT PDO Receive  Priority=2  sig_name=Drive 3 (C1150-DS-XC-0S).Cylic Mode Inputs.Position actual value (units)  sig_offset=1048  sig_type=int32  type_size=32  sig_dim=1  device_id=0  sample_time=0.001000
      settings: SourceProductBaseCode=XP
  Position Actual Value4 : xpcethercatlib/EtherCAT PDO Receive  Priority=2  sig_name=Drive 4 (C1150-DS-XC-0S).Cylic Mode Inputs.Position actual value (units)  sig_offset=1208  sig_type=int32  type_size=32  sig_dim=1  device_id=0  sample_time=0.001000
      settings: SourceProductBaseCode=XP
  Position Actual Value5 : xpcethercatlib/EtherCAT PDO Receive  Priority=2  sig_name=Drive 5 (C1150-DS-XC-0S).Cylic Mode Inputs.Position actual value (units)  sig_offset=1368  sig_type=int32  type_size=32  sig_dim=1  device_id=0  sample_time=0.001000
      settings: SourceProductBaseCode=XP
  Position Actual Value6 : xpcethercatlib/EtherCAT PDO Receive  Priority=2  sig_name=Drive 6 (C1150-DS-XC-0S).Cylic Mode Inputs.Position actual value (units)  sig_offset=1528  sig_type=int32  type_size=32  sig_dim=1  device_id=0  sample_time=0.001000
      settings: SourceProductBaseCode=XP
  Position Actual Value7 : xpcethercatlib/EtherCAT PDO Receive  Priority=2  sig_name=Drive 7 (C1150-DS-XC-0S).Cylic Mode Inputs.Position actual value (units)  sig_offset=1688  sig_type=int32  type_size=32  sig_dim=1  device_id=0  sample_time=0.001000
      settings: SourceProductBaseCode=XP
  Position Actual Value8 : xpcethercatlib/EtherCAT PDO Receive  Priority=2  sig_name=Drive 8 (C1150-DS-XC-0S).Cylic Mode Inputs.Position actual value (units)  sig_offset=1848  sig_type=int32  type_size=32  sig_dim=1  device_id=0  sample_time=0.001000
      settings: SourceProductBaseCode=XP
  Ticks to mm : Gain  Gain=1/10000
  Actual Position : Outport
  wires:
  Position Actual Value2/1 -> Mux6/2  "Actual Position"
  Position Actual Value4/1 -> Mux6/4  "Actual Position"
  Position Actual Value1/1 -> Mux6/1  "Actual Position"
  Position Actual Value3/1 -> Mux6/3  "Actual Position"
  Position Actual Value7/1 -> Mux6/7  "Actual Position"
  Position Actual Value6/1 -> Mux6/6  "Actual Position"
  Position Actual Value8/1 -> Mux6/8  "Actual Position"
  Position Actual Value5/1 -> Mux6/5  "Actual Position"
  Ticks to mm/1 -> Cast To Double2/1
  Cast To Double2/1 -> Actual Position/1  "Actual Position"
  Mux6/1 -> Ticks to mm/1  "Actual Position"

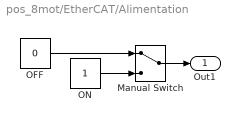
== system pos_8mot/EtherCAT/Alimentation ==
  Manual Switch : ManualSwitch
  OFF : Constant  Value=0
  ON : Constant
  Out1 : Outport
  wires:
  OFF/1 -> Manual Switch/1
  ON/1 -> Manual Switch/2
  Manual Switch/1 -> Out1/1

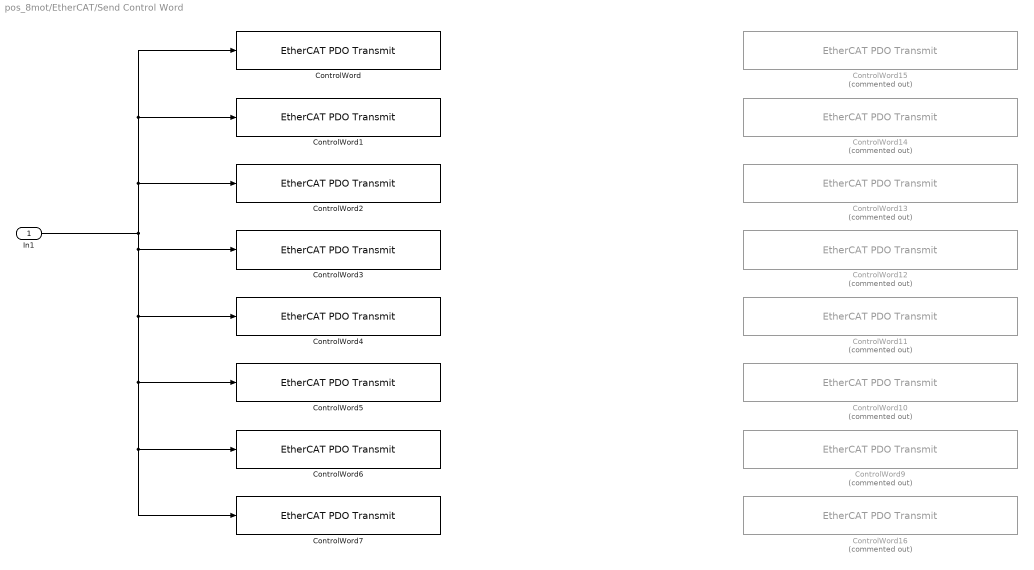
== system pos_8mot/EtherCAT/Send Control Word ==
  In1 : Inport
  ControlWord : xpcethercatlib/EtherCAT PDO Transmit   Priority=3  sig_name=Drive 1 (C1150-DS-XC-0S).Cylic Position Mode.Controlword  sig_offset=696  sig_type=uint16  type_size=16  sig_dim=1  device_id=0  sample_time=0.001000
      settings: SourceProductBaseCode=XP
  ControlWord1 : xpcethercatlib/EtherCAT PDO Transmit   Priority=3  sig_name=Drive 2 (C1150-DS-XC-0S).Cylic Position Mode.Controlword  sig_offset=872  sig_type=uint16  type_size=16  sig_dim=1  device_id=0  sample_time=0.001000
      settings: SourceProductBaseCode=XP
  ControlWord10 : xpcethercatlib/EtherCAT PDO Transmit   Priority=3  Commented=on  sig_name=Drive 6 (C1150-DS-XC-0S).Cylic Position Velocity Mode.Controlword  sig_offset=1432  sig_type=uint16  type_size=16  sig_dim=1  device_id=0  sample_time=0.001000
      settings: SourceProductBaseCode=XP
  ControlWord11 : xpcethercatlib/EtherCAT PDO Transmit   Priority=3  Commented=on  sig_name=Drive 5 (C1150-DS-XC-0S).Cylic Position Velocity Mode.Controlword  sig_offset=1288  sig_type=uint16  type_size=16  sig_dim=1  device_id=0  sample_time=0.001000
      settings: SourceProductBaseCode=XP
  ControlWord12 : xpcethercatlib/EtherCAT PDO Transmit   Priority=3  Commented=on  sig_name=Drive 4 (C1150-DS-XC-0S).Cylic Position Velocity Mode.Controlword  sig_offset=1144  sig_type=uint16  type_size=16  sig_dim=1  device_id=0  sample_time=0.001000
      settings: SourceProductBaseCode=XP
  ControlWord13 : xpcethercatlib/EtherCAT PDO Transmit   Priority=3  Commented=on  sig_name=Drive 3 (C1150-DS-XC-0S).Cylic Position Velocity Mode.Controlword  sig_offset=1000  sig_type=uint16  type_size=16  sig_dim=1  device_id=0  sample_time=0.001000
      settings: SourceProductBaseCode=XP
  ControlWord14 : xpcethercatlib/EtherCAT PDO Transmit   Priority=3  Commented=on  sig_name=Drive 2 (C1150-DS-XC-0S).Cylic Position Velocity Mode.Controlword  sig_offset=856  sig_type=uint16  type_size=16  sig_dim=1  device_id=0  sample_time=0.001000
      settings: SourceProductBaseCode=XP
  ControlWord15 : xpcethercatlib/EtherCAT PDO Transmit   Priority=3  Commented=on  sig_name=Drive 1 (C1150-DS-XC-0S).Cylic Position Velocity Mode.Controlword  sig_offset=696  sig_type=uint16  type_size=16  sig_dim=1  device_id=0  sample_time=0.001000
      settings: SourceProductBaseCode=XP
  ControlWord16 : xpcethercatlib/EtherCAT PDO Transmit   Priority=3  Commented=on  sig_name=Drive 8 (C1150-DS-XC-0S).Cylic Position Velocity Mode.Controlword  sig_offset=1720  sig_type=uint16  type_size=16  sig_dim=1  device_id=0  sample_time=0.001000
      settings: SourceProductBaseCode=XP
  ControlWord2 : xpcethercatlib/EtherCAT PDO Transmit   Priority=3  sig_name=Drive 3 (C1150-DS-XC-0S).Cylic Position Mode.Controlword  sig_offset=1032  sig_type=uint16  type_size=16  sig_dim=1  device_id=0  sample_time=0.001000
      settings: SourceProductBaseCode=XP
  ControlWord3 : xpcethercatlib/EtherCAT PDO Transmit   Priority=3  sig_name=Drive 4 (C1150-DS-XC-0S).Cylic Position Mode.Controlword  sig_offset=1192  sig_type=uint16  type_size=16  sig_dim=1  device_id=0  sample_time=0.001000
      settings: SourceProductBaseCode=XP
  ControlWord4 : xpcethercatlib/EtherCAT PDO Transmit   Priority=3  sig_name=Drive 5 (C1150-DS-XC-0S).Cylic Position Mode.Controlword  sig_offset=1352  sig_type=uint16  type_size=16  sig_dim=1  device_id=0  sample_time=0.001000
      settings: SourceProductBaseCode=XP
  ControlWord5 : xpcethercatlib/EtherCAT PDO Transmit   Priority=3  sig_name=Drive 6 (C1150-DS-XC-0S).Cylic Position Mode.Controlword  sig_offset=1512  sig_type=uint16  type_size=16  sig_dim=1  device_id=0  sample_time=0.001000
      settings: SourceProductBaseCode=XP
  ControlWord6 : xpcethercatlib/EtherCAT PDO Transmit   Priority=3  sig_name=Drive 7 (C1150-DS-XC-0S).Cylic Position Mode.Controlword  sig_offset=1672  sig_type=uint16  type_size=16  sig_dim=1  device_id=0  sample_time=0.001000
      settings: SourceProductBaseCode=XP
  ControlWord7 : xpcethercatlib/EtherCAT PDO Transmit   Priority=3  sig_name=Drive 8 (C1150-DS-XC-0S).Cylic Position Mode.Controlword  sig_offset=1832  sig_type=uint16  type_size=16  sig_dim=1  device_id=0  sample_time=0.001000
      settings: SourceProductBaseCode=XP
  ControlWord9 : xpcethercatlib/EtherCAT PDO Transmit   Priority=3  Commented=on  sig_name=Drive 7 (C1150-DS-XC-0S).Cylic Position Velocity Mode.Controlword  sig_offset=1576  sig_type=uint16  type_size=16  sig_dim=1  device_id=0  sample_time=0.001000
      settings: SourceProductBaseCode=XP
  wires:
  In1/1 -> ControlWord2/1, ControlWord1/1, ControlWord/1, ControlWord7/1, ControlWord6/1, ControlWord5/1, ControlWord4/1, ControlWord3/1

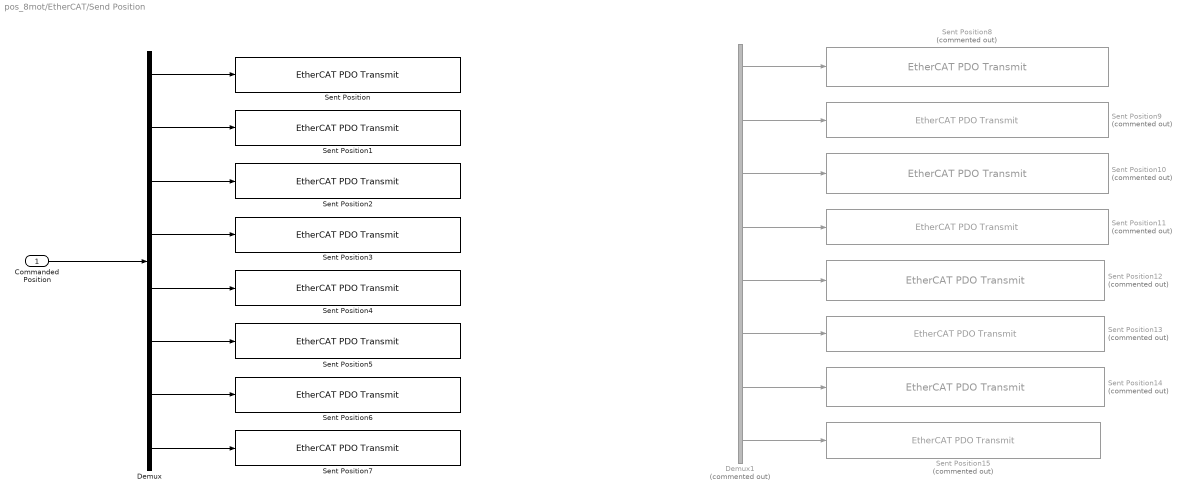
== system pos_8mot/EtherCAT/Send Position ==
  Commanded Position : Inport
  Demux : Demux  Outputs=8
  Demux1 : Demux  Commented=on  Outputs=8
  Sent Position : xpcethercatlib/EtherCAT PDO Transmit   Priority=3  sig_name=Drive 1 (C1150-DS-XC-0S).Cylic Position Mode.Target position  sig_offset=712  sig_type=int32  type_size=32  sig_dim=1  device_id=0  sample_time=0.001000
      settings: SourceProductBaseCode=XP
  Sent Position1 : xpcethercatlib/EtherCAT PDO Transmit   Priority=3  sig_name=Drive 2 (C1150-DS-XC-0S).Cylic Position Mode.Target position  sig_offset=888  sig_type=int32  type_size=32  sig_dim=1  device_id=0  sample_time=0.001000
      settings: SourceProductBaseCode=XP
  Sent Position10 : xpcethercatlib/EtherCAT PDO Transmit   Priority=3  Commented=on  sig_name=Drive 3 (C1150-DS-XC-0S).Cylic Position Velocity Mode.Target position  sig_offset=1016  sig_type=int32  type_size=32  sig_dim=1  device_id=0  sample_time=0.001000
      settings: SourceProductBaseCode=XP
  Sent Position11 : xpcethercatlib/EtherCAT PDO Transmit   Priority=3  Commented=on  sig_name=Drive 4 (C1150-DS-XC-0S).Cylic Position Velocity Mode.Target position  sig_offset=1160  sig_type=int32  type_size=32  sig_dim=1  device_id=0  sample_time=0.001000
      settings: SourceProductBaseCode=XP
  Sent Position12 : xpcethercatlib/EtherCAT PDO Transmit   Priority=3  Commented=on  sig_name=Drive 5 (C1150-DS-XC-0S).Cylic Position Velocity Mode.Target position  sig_offset=1304  sig_type=int32  type_size=32  sig_dim=1  device_id=0  sample_time=0.001000
      settings: SourceProductBaseCode=XP
  Sent Position13 : xpcethercatlib/EtherCAT PDO Transmit   Priority=3  Commented=on  sig_name=Drive 6 (C1150-DS-XC-0S).Cylic Position Velocity Mode.Target position  sig_offset=1448  sig_type=int32  type_size=32  sig_dim=1  device_id=0  sample_time=0.001000
      settings: SourceProductBaseCode=XP
  Sent Position14 : xpcethercatlib/EtherCAT PDO Transmit   Priority=3  Commented=on  sig_name=Drive 7 (C1150-DS-XC-0S).Cylic Position Velocity Mode.Target position  sig_offset=1592  sig_type=int32  type_size=32  sig_dim=1  device_id=0  sample_time=0.001000
      settings: SourceProductBaseCode=XP
  Sent Position15 : xpcethercatlib/EtherCAT PDO Transmit   Priority=3  Commented=on  sig_name=Drive 8 (C1150-DS-XC-0S).Cylic Position Velocity Mode.Target position  sig_offset=1736  sig_type=int32  type_size=32  sig_dim=1  device_id=0  sample_time=0.001000
      settings: SourceProductBaseCode=XP
  Sent Position2 : xpcethercatlib/EtherCAT PDO Transmit   Priority=3  sig_name=Drive 3 (C1150-DS-XC-0S).Cylic Position Mode.Target position  sig_offset=1048  sig_type=int32  type_size=32  sig_dim=1  device_id=0  sample_time=0.001000
      settings: SourceProductBaseCode=XP
  Sent Position3 : xpcethercatlib/EtherCAT PDO Transmit   Priority=3  sig_name=Drive 4 (C1150-DS-XC-0S).Cylic Position Mode.Target position  sig_offset=1208  sig_type=int32  type_size=32  sig_dim=1  device_id=0  sample_time=0.001000
      settings: SourceProductBaseCode=XP
  Sent Position4 : xpcethercatlib/EtherCAT PDO Transmit   Priority=3  sig_name=Drive 5 (C1150-DS-XC-0S).Cylic Position Mode.Target position  sig_offset=1368  sig_type=int32  type_size=32  sig_dim=1  device_id=0  sample_time=0.001000
      settings: SourceProductBaseCode=XP
  Sent Position5 : xpcethercatlib/EtherCAT PDO Transmit   Priority=3  sig_name=Drive 6 (C1150-DS-XC-0S).Cylic Position Mode.Target position  sig_offset=1528  sig_type=int32  type_size=32  sig_dim=1  device_id=0  sample_time=0.001000
      settings: SourceProductBaseCode=XP
  Sent Position6 : xpcethercatlib/EtherCAT PDO Transmit   Priority=3  sig_name=Drive 7 (C1150-DS-XC-0S).Cylic Position Mode.Target position  sig_offset=1688  sig_type=int32  type_size=32  sig_dim=1  device_id=0  sample_time=0.001000
      settings: SourceProductBaseCode=XP
  Sent Position7 : xpcethercatlib/EtherCAT PDO Transmit   Priority=3  sig_name=Drive 8 (C1150-DS-XC-0S).Cylic Position Mode.Target position  sig_offset=1848  sig_type=int32  type_size=32  sig_dim=1  device_id=0  sample_time=0.001000
      settings: SourceProductBaseCode=XP
  Sent Position8 : xpcethercatlib/EtherCAT PDO Transmit   Priority=3  Commented=on  sig_name=Drive 1 (C1150-DS-XC-0S).Cylic Position Velocity Mode.Target position  sig_offset=712  sig_type=int32  type_size=32  sig_dim=1  device_id=0  sample_time=0.001000
      settings: SourceProductBaseCode=XP
  Sent Position9 : xpcethercatlib/EtherCAT PDO Transmit   Priority=3  Commented=on  sig_name=Drive 2 (C1150-DS-XC-0S).Cylic Position Velocity Mode.Target position  sig_offset=872  sig_type=int32  type_size=32  sig_dim=1  device_id=0  sample_time=0.001000
      settings: SourceProductBaseCode=XP
  wires:
  Demux/1 -> Sent Position/1
  Demux/2 -> Sent Position1/1
  Demux/3 -> Sent Position2/1
  Demux/4 -> Sent Position3/1
  Demux/5 -> Sent Position4/1
  Demux/6 -> Sent Position5/1
  Demux/7 -> Sent Position6/1
  Demux/8 -> Sent Position7/1
  Demux1/7 -> Sent Position14/1
  Demux1/6 -> Sent Position13/1
  Demux1/3 -> Sent Position10/1
  Demux1/4 -> Sent Position11/1
  Demux1/2 -> Sent Position9/1
  Demux1/8 -> Sent Position15/1
  Demux1/5 -> Sent Position12/1
  Demux1/1 -> Sent Position8/1
  Commanded Position/1 -> Demux/1
